simulink model "SF015A_WhlImbRejctn"  (R2013b)
settings: Solver=FixedStepDiscrete  SolverMode=SingleTasking  StartTime=0.0  StopTime=1  FixedStep=0.002  RelTol=1e-3
values from neighbouring files (symbols this model uses):
  ACTIVBANDMAX_ULS_U32 = DataDict.Constant    [SF015A_WhlImbRejctn_DataDict.m]
  ADAPVFILMAX_ULS_F32 = DataDict.Constant    [SF015A_WhlImbRejctn_DataDict.m]
  ARCHGLBPRM_180OVERPI_ULS_F32 = DataDict.Constant    [SF015A_WhlImbRejctn_DataDict.m]
  ARCHGLBPRM_2MILLISEC_SEC_F32 = DataDict.Constant    [SF015A_WhlImbRejctn_DataDict.m]
  ARCHGLBPRM_2PI_ULS_F32 = DataDict.Constant    [SF015A_WhlImbRejctn_DataDict.m]
  ARCHGLBPRM_FLOATZEROTHD_ULS_F32 = DataDict.Constant    [SF015A_WhlImbRejctn_DataDict.m]
  ARCHGLBPRM_PI_ULS_F32 = DataDict.Constant    [SF015A_WhlImbRejctn_DataDict.m]
  ARCHGLBPRM_PIOVER180_ULS_F32 = DataDict.Constant    [SF015A_WhlImbRejctn_DataDict.m]
  ARCHGLBPRM_PIOVER2_ULS_F32 = DataDict.Constant    [SF015A_WhlImbRejctn_DataDict.m]
  CALMINSPERCOUNT_ULS_F32 = DataDict.Constant    [SF015A_WhlImbRejctn_DataDict.m]
  DURATIONDISABLE_CNT_U16 = DataDict.Constant    [SF015A_WhlImbRejctn_DataDict.m]
  FILTWHLSPDMAX_MOTRADPERSEC_F32 = DataDict.Constant    [SF015A_WhlImbRejctn_DataDict.m]
  MICROSECTOMILLISEC_ULS_F32 = DataDict.Constant    [SF015A_WhlImbRejctn_DataDict.m]
  MINSTOMILLISEC_ULS_F32 = DataDict.Constant    [SF015A_WhlImbRejctn_DataDict.m]
  NINETY_ULS_F32 = DataDict.Constant    [SF015A_WhlImbRejctn_DataDict.m]
  NODEBSTEP_CNT_U16 = DataDict.Constant    [SF015A_WhlImbRejctn_DataDict.m]
  NROFDLY_CNT_U08 = DataDict.Constant    [SF015A_WhlImbRejctn_DataDict.m]
  ONEHALF_ULS_F32 = DataDict.Constant    [SF015A_WhlImbRejctn_DataDict.m]
  ONEHUNDRED_ULS_F32 = DataDict.Constant    [SF015A_WhlImbRejctn_DataDict.m]
  ONEOVRTHREE_ULS_F32 = DataDict.Constant    [SF015A_WhlImbRejctn_DataDict.m]
  ONEOVRTWENTY_ULS_F32 = DataDict.Constant    [SF015A_WhlImbRejctn_DataDict.m]
  ONETHOUSAND_ULS_F32 = DataDict.Constant    [SF015A_WhlImbRejctn_DataDict.m]
  PEAKMAX_ULS_F32 = DataDict.Constant    [SF015A_WhlImbRejctn_DataDict.m]
  PEAKMIN_ULS_F32 = DataDict.Constant    [SF015A_WhlImbRejctn_DataDict.m]
  PHAADJMAX_ULS_F32 = DataDict.Constant    [SF015A_WhlImbRejctn_DataDict.m]
  PITIMESSAMPLETIME_ULS_F32 = DataDict.Constant    [SF015A_WhlImbRejctn_DataDict.m]
  STOREDMINSPERCOUNT_ULS_F32 = DataDict.Constant    [SF015A_WhlImbRejctn_DataDict.m]
  TWO_ULS_F32 = DataDict.Constant    [SF015A_WhlImbRejctn_DataDict.m]
  TWOOVRTHREE_ULS_F32 = DataDict.Constant    [SF015A_WhlImbRejctn_DataDict.m]
  WhlImbRejctnAdpvFac = DataDict.Calibration    [SF015A_WhlImbRejctn_DataDict.m]
  WhlImbRejctnAutScaEna = DataDict.Calibration    [SF015A_WhlImbRejctn_DataDict.m]
  WhlImbRejctnAutScaTar = DataDict.Calibration    [SF015A_WhlImbRejctn_DataDict.m]
  WhlImbRejctnCurrMgnSlewPerLoop = DataDict.Calibration    [SF015A_WhlImbRejctn_DataDict.m]
  WhlImbRejctnDcTrendFltRcvryDly = DataDict.Calibration    [SF015A_WhlImbRejctn_DataDict.m]
  WhlImbRejctnDcTrendFltRcvryNegStep = DataDict.Calibration    [SF015A_WhlImbRejctn_DataDict.m]
  WhlImbRejctnDcTrendFltRcvryPosStep = DataDict.Calibration    [SF015A_WhlImbRejctn_DataDict.m]
  WhlImbRejctnDcTrendFltRcvryThd = DataDict.Calibration    [SF015A_WhlImbRejctn_DataDict.m]
  WhlImbRejctnDcTrendTh2Tq = DataDict.Calibration    [SF015A_WhlImbRejctn_DataDict.m]
  WhlImbRejctnDcTrendThTq = DataDict.Calibration    [SF015A_WhlImbRejctn_DataDict.m]
  WhlImbRejctnDcTrendTi2Sec = DataDict.Calibration    [SF015A_WhlImbRejctn_DataDict.m]
  WhlImbRejctnDcTrendTiSec = DataDict.Calibration    [SF015A_WhlImbRejctn_DataDict.m]
  WhlImbRejctnEnaSlewPerLoop = DataDict.Calibration    [SF015A_WhlImbRejctn_DataDict.m]
  WhlImbRejctnFctEna = DataDict.Calibration    [SF015A_WhlImbRejctn_DataDict.m]
  WhlImbRejctnFrqDiagcAmpThd = DataDict.Calibration    [SF015A_WhlImbRejctn_DataDict.m]
  WhlImbRejctnFrqDiagcEna = DataDict.Calibration    [SF015A_WhlImbRejctn_DataDict.m]
  WhlImbRejctnFrqDiagcFltRcvryDly = DataDict.Calibration    [SF015A_WhlImbRejctn_DataDict.m]
  WhlImbRejctnFrqDiagcFltRcvryNegStep = DataDict.Calibration    [SF015A_WhlImbRejctn_DataDict.m]
  WhlImbRejctnFrqDiagcFltRcvryPosStep = DataDict.Calibration    [SF015A_WhlImbRejctn_DataDict.m]
  WhlImbRejctnFrqDiagcFltRcvryThd = DataDict.Calibration    [SF015A_WhlImbRejctn_DataDict.m]
  WhlImbRejctnFrqDiagcThd = DataDict.Calibration    [SF015A_WhlImbRejctn_DataDict.m]
  WhlImbRejctnFrqDiagcTout = DataDict.Calibration    [SF015A_WhlImbRejctn_DataDict.m]
  WhlImbRejctnFrqDiagcUgrPoleMgn = DataDict.Calibration    [SF015A_WhlImbRejctn_DataDict.m]
  WhlImbRejctnFrqScaTblX = DataDict.Calibration    [SF015A_WhlImbRejctn_DataDict.m]
  WhlImbRejctnMaxDurn = DataDict.Calibration    [SF015A_WhlImbRejctn_DataDict.m]
  WhlImbRejctnMaxMgn = DataDict.Calibration    [SF015A_WhlImbRejctn_DataDict.m]
  WhlImbRejctnMaxMgnFltNegStep = DataDict.Calibration    [SF015A_WhlImbRejctn_DataDict.m]
  WhlImbRejctnMaxMgnFltPosStep = DataDict.Calibration    [SF015A_WhlImbRejctn_DataDict.m]
  WhlImbRejctnMaxMgnFltRcvryDly = DataDict.Calibration    [SF015A_WhlImbRejctn_DataDict.m]
  WhlImbRejctnMaxMgnFltRcvryNegStep = DataDict.Calibration    [SF015A_WhlImbRejctn_DataDict.m]
  WhlImbRejctnMaxMgnFltRcvryPosStep = DataDict.Calibration    [SF015A_WhlImbRejctn_DataDict.m]
  WhlImbRejctnMaxMgnFltRcvryThd = DataDict.Calibration    [SF015A_WhlImbRejctn_DataDict.m]
  WhlImbRejctnMaxMgnFltThd = DataDict.Calibration    [SF015A_WhlImbRejctn_DataDict.m]
  WhlImbRejctnMgnEstimnDeltaSca = DataDict.Calibration    [SF015A_WhlImbRejctn_DataDict.m]
  WhlImbRejctnMgnEstimnDiThd = DataDict.Calibration    [SF015A_WhlImbRejctn_DataDict.m]
  WhlImbRejctnMgnEstimnEnaThd = DataDict.Calibration    [SF015A_WhlImbRejctn_DataDict.m]
  WhlImbRejctnMgnEstimnFrq = DataDict.Calibration    [SF015A_WhlImbRejctn_DataDict.m]
  WhlImbRejctnMgnEstimnFrqDelta = DataDict.Calibration    [SF015A_WhlImbRejctn_DataDict.m]
  WhlImbRejctnMgnEstimnLeak = DataDict.Calibration    [SF015A_WhlImbRejctn_DataDict.m]
  WhlImbRejctnRampDwnTi = DataDict.Calibration    [SF015A_WhlImbRejctn_DataDict.m]
  WhlImbRejctnScaCncl = DataDict.Calibration    [SF015A_WhlImbRejctn_DataDict.m]
  WhlImbRejctnUgrPoleMgn = DataDict.Calibration    [SF015A_WhlImbRejctn_DataDict.m]
  WhlImbRejctnVehSpdEna = DataDict.Calibration    [SF015A_WhlImbRejctn_DataDict.m]
  WhlImbRejctnWhlSpdCorrlnFltRcvryDly = DataDict.Calibration    [SF015A_WhlImbRejctn_DataDict.m]
  WhlImbRejctnWhlSpdCorrlnFltRcvryNegStep = DataDict.Calibration    [SF015A_WhlImbRejctn_DataDict.m]
  WhlImbRejctnWhlSpdCorrlnFltRcvryPosStep = DataDict.Calibration    [SF015A_WhlImbRejctn_DataDict.m]
  WhlImbRejctnWhlSpdCorrlnFltRcvryThd = DataDict.Calibration    [SF015A_WhlImbRejctn_DataDict.m]
  WhlImbRejctnWhlSpdCorrlnThd = DataDict.Calibration    [SF015A_WhlImbRejctn_DataDict.m]
  WhlImbRejctnWhlSpdCorrlnTi = DataDict.Calibration    [SF015A_WhlImbRejctn_DataDict.m]
  WIRCMDMAX_MOTNWTMTR_F32 = DataDict.Constant    [SF015A_WhlImbRejctn_DataDict.m]
  ZERO_ULS_F32 = DataDict.Constant    [SF015A_WhlImbRejctn_DataDict.m]
undefined symbols (not defined in the file or in its folder): Cntr, NtcNr1, NvmGetErrSts1, SigQlfr1, Sts, SysSt1
libraries: simulink x32, FixdToFloat x32, Fil x20, NxtrLim x15, NxtrNvM x12, NxtrAbslt x8, NxtrMath x7, NxtrMax x6, NxtrMin x4, FloatToFixd x2, LnrIntrpn x2, NxtrSign x1
(part 4 of 12)

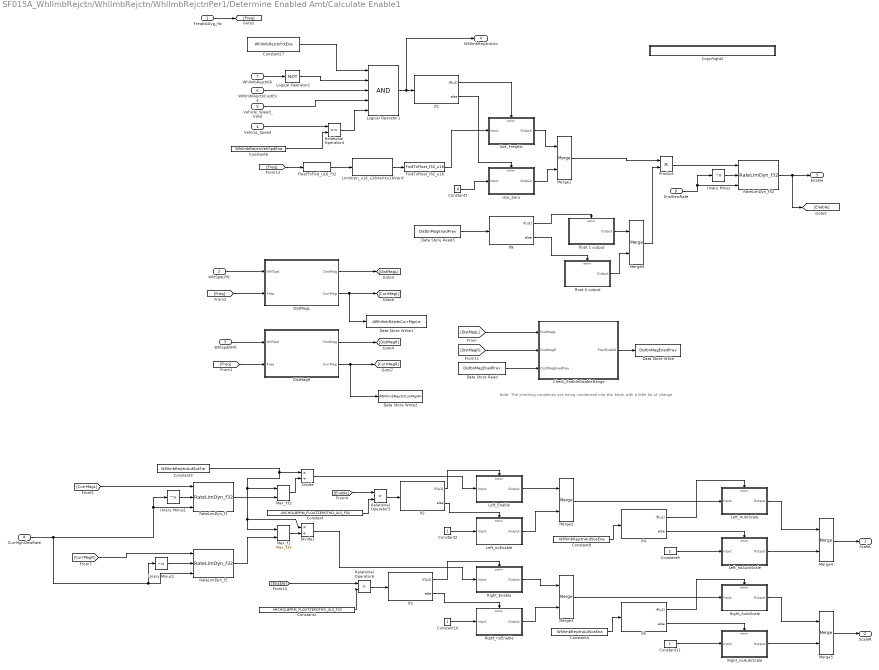
== system SF015A_WhlImbRejctn/WhlImbRejctn/WhlImbRejctnPer1/Determine Enabled Amt/Calculate Enable1 ==
  note: Note: The checking conditions are being condensed into thsi block with a little bit of change
  FreqEstAvg_Hz : Inport
  WhlSpdLFilt : Inport  Port=2
  WhlSpdRFilt : Inport  Port=3
  Vehicle_Speed : Inport  Port=4
  Vehicle_Speed_Valid : Inport  Port=5
  WhlImbRejctnCustEna : Inport  Port=6
  WhlImbRejctnDi : Inport  Port=7
  CurrMgnSlewRate : Inport  Port=8
  EnaSlewRate : Inport  Port=9
  Check_EnableDisableRange : Subsystem
  Constant : Constant  Value=ARCHGLBPRM_FLOATZEROTHD_ULS_F32
  Constant1 : Constant  Value=ARCHGLBPRM_FLOATZEROTHD_ULS_F32
  Constant{2,9..11} (4 alike) : Constant  OutDataTypeStr=single
  Constant17 : Constant  Value=WhlImbRejctnFctEna
  Constant3 : Constant  Value=WhlImbRejctnAutScaTar
  Constant4 : Constant  Value=WhlImbRejctnAutScaEna
  Constant6 : Constant  Value=WhlImbRejctnVehSpdEna
  Constant7 : Constant  Value=0  OutDataTypeStr=single
  Constant8 : Constant  Value=WhlImbRejctnAutScaEna
  CopyRight2 : Subsystem  Description=|  mask(Copyright Information){none=on}
      | Copyright info block.                                               
      |                                                                     
      | Place copyright information at the top of every subsystem in design.
      mask prompts: none "No parameters"
      mask help: Place copyright information at the top of every subsystem in design.
      mask Display:
      | NxtrConf = 'Nexteer Confidential';
      | 
      | sys = bdroot; %handle for the current model ("system")
      | first = get_param(sys,'Created');
      | first = first(end-3:end);  %year is last four digits
      | 
      | last = get_param(sys,'LastModifiedDate');
      | if isempty(last)
      |     last = datestr(now,'yyyy');
      | else
      |     last = last(end-3:end);
      | end
      | 
      | if strcmp(first,last)
      |     fprintf('%s -- Copyright %s Nexteer',NxtrConf,first)
      | else
      |     fprintf('%s -- %s%s- %s Nexteer',NxtrConf,char(169),first,last)
      | end
  Data Store Read : DataStoreRead  Priority=2  DataStoreName=DistbnMagEnadPrev
      settings: AttributesFormatString=Priority=%<Priority>
  Data Store Read3 : DataStoreRead  Priority=1  DataStoreName=DistbnMagEnadPrev
      settings: AttributesFormatString=Priority=%<Priority>
  Data Store Write : DataStoreWrite  Priority=3  DataStoreName=DistbnMagEnadPrev
      settings: AttributesFormatString=Priority=%<Priority>
  Data Store Write1 : DataStoreWrite  DataStoreName=dWhlImbRejctnCurrMgnLe
  Data Store Write2 : DataStoreWrite  DataStoreName=dWhlImbRejctnCurrMgnRi
  DistMagL : Subsystem
  DistMagR : Subsystem
  Divide : Product  Inputs=*/
  Divide1 : Product  Inputs=*/
  FixdToFloat_f32_u16 : FixdToFloat/FixdToFloat_f32_u16  Param1=0
  FloatToFixd_u16_f32 : FloatToFixd/FloatToFixd_u16_f32  Param1=0
  If1 : If  RequirementInfo={} %GIDa_7d8297b8_b265_4b47_b8b2_192e5a92e4fb  IfExpression=u1
  If2 : If  RequirementInfo={} %GIDa_0556d171_7866_4516_8d40_956f321be7bc  IfExpression=u1
  If3 : If  RequirementInfo={} %GIDa_fcbce161_0599_4b7a_b23c_d7b8d7e27a0f  IfExpression=u1
  If4 : If  RequirementInfo={} %GIDa_46a5a10e_d4b7_40a4_ac58_d797cb624c83  IfExpression=u1
  If5 : If  RequirementInfo={} %GIDa_3e7d8d50_75ba_4493_bb61_e3ba5f1e5c7c  IfExpression=u1
  If9 : If  RequirementInfo={} %GIDa_220c56c6_5b09_48da_a4b3_63431d3edf67  IfExpression=u1
  Left_AutoScale : Subsystem  RequirementInfo={} %GIDa_9c3ac42f_cbc1_49be_98f6_7ec1737ed2ed  TreatAsAtomicUnit=on
  Left_Enable : Subsystem  RequirementInfo={} %GIDa_d65479b8_5b54_4e68_bf36_3b31ad24537e  TreatAsAtomicUnit=on
  Left_noAutoScale : Subsystem  RequirementInfo={} %GIDa_bdc4660b_a72c_40f0_89ba_28a8acc1db11  TreatAsAtomicUnit=on
  Left_noEnable : Subsystem  RequirementInfo={} %GIDa_18e28b2f_1f1d_4076_8343_147cb5570336  TreatAsAtomicUnit=on
  LnrIntrpn_u16_u16VariXu16VariY : LnrIntrpn/LnrIntrpn_u16_u16VariXu16VariY  XTbl=WhlImbRejctnFrqScaTblX  YTbl=WhlImbRejctnFrqScaTblY
      settings: AttributesFormatString=Lnr ( u16VariX , u16VariY )
  Logical Operator1 : Logic  Inputs=5  AllPortsSameDT=off  OutDataTypeStr=boolean
  Logical Operator2 : Logic  Operator=NOT  Inputs=5  AllPortsSameDT=off  OutDataTypeStr=boolean
  Max_f1 : NxtrMax/Max_f32  SFunctionSpec=single y1 = Max_f32(single u1, single u2)
      settings: AttributesFormatString=%<Name>
  Max_f32 : NxtrMax/Max_f32  SFunctionSpec=single y1 = Max_f32(single u1, single u2)
      settings: AttributesFormatString=%<Name>
  Merge{1..5,9} (6 alike) : Merge
  Product : Product
  RateLimDyn_f1 : NxtrLim/RateLimDyn_f32  StVar=LeCurrMgnSlewPerLoop  Ts=ARCHGLBPRM_2MILLISEC_SEC_F32
      settings: AttributesFormatString=StVar: %<StVar>
  RateLimDyn_f2 : NxtrLim/RateLimDyn_f32  StVar=RiCurrMgnSlewPerLoop  Ts=ARCHGLBPRM_2MILLISEC_SEC_F32
      settings: AttributesFormatString=StVar: %<StVar>
  RateLimDyn_f32 : NxtrLim/RateLimDyn_f32  StVar=EnaSlewPerLoop  Ts=ARCHGLBPRM_2MILLISEC_SEC_F32
      settings: AttributesFormatString=StVar: %<StVar>
  Relational Operator4 : RelationalOperator  OutDataTypeStr=boolean
  Relational Operator5 : RelationalOperator  Operator=>  OutDataTypeStr=boolean
  Relational Operator6 : RelationalOperator  Operator=>  OutDataTypeStr=boolean
  Right_AutoScale : Subsystem  RequirementInfo={} %GIDa_13da9aa5_5c49_428f_b287_6188729282ed  TreatAsAtomicUnit=on
  Right_Enable : Subsystem  RequirementInfo={} %GIDa_75bbbddb_2767_47a3_9165_63797ed0e216  TreatAsAtomicUnit=on
  Right_noAutoScale : Subsystem  RequirementInfo={} %GIDa_e3eec680_517e_4da7_948a_b3f8124b2971  TreatAsAtomicUnit=on
  Right_noEnable : Subsystem  RequirementInfo={} %GIDa_b2607bc0_d58b_406c_8b11_3dee4f11cd4c  TreatAsAtomicUnit=on
  Unary Minus : UnaryMinus
  Unary Minus1 : UnaryMinus
  Unary Minus2 : UnaryMinus
  Use_FreqEst : Subsystem  RequirementInfo={} %GIDa_066b3e73_a3fa_4d6c_9937_967fb698f328  TreatAsAtomicUnit=on
  Use_Zero : Subsystem  RequirementInfo={} %GIDa_7b829dcd_761e_44e8_86d6_74abc0632468  TreatAsAtomicUnit=on
  float 0 output : Subsystem  RequirementInfo={} %GIDa_73b9442c_5069_415a_a71a_08570183037e  TreatAsAtomicUnit=on
  float 1 output : Subsystem  RequirementInfo={} %GIDa_eb48623e_e509_47ed_bd29_5bcb251c6a65  TreatAsAtomicUnit=on
  ScaleL : Outport
  ScaleR : Outport  Port=2
  Enable : Outport  Port=3
  WhlImbRejctnActv : Outport  Port=4
  wires:
  FreqEstAvg_Hz/1 -> [Freq]
  WhlSpdLFilt/1 -> DistMagL/1(WhlSpd)
  [Freq] -> DistMagL/2(Freq)
  WhlSpdRFilt/1 -> DistMagR/1(WhlSpd)
  [Freq] -> DistMagR/2(Freq)
  DistMagL/1(DistMag) -> [DistMagL]
  DistMagR/1(DistMag) -> [DistMagR]
  Data Store Read3/1 -> If9/1
  Constant3/1 -> Max_f32/1, Max_f1/1, Divide1/1, Divide/1
  DistMagL/2(CurrMag) -> Data Store Write1/1, [CurrMagL]
  DistMagR/2(CurrMag) -> Data Store Write2/1, [CurrMagR]
  Max_f32/1 -> Divide/2
  [CurrMagL] -> RateLimDyn_f1/1
  Max_f1/1 -> Divide1/2
  [CurrMagR] -> RateLimDyn_f2/1
  Vehicle_Speed/1 -> Relational Operator4/1
  Constant6/1 -> Relational Operator4/2
  Relational Operator4/1 -> Logical Operator1/5
  Vehicle_Speed_Valid/1 -> Logical Operator1/4
  WhlImbRejctnCustEna/1 -> Logical Operator1/3
  WhlImbRejctnDi/1 -> Logical Operator2/1
  Constant7/1 -> Use_Zero/1(Input)
  If1/1 -> Use_FreqEst/Action
  If1/2 -> Use_Zero/Action
  Logical Operator1/1 -> WhlImbRejctnActv/1, If1/1
  Use_FreqEst/1(Output) -> Merge1/1
  Use_Zero/1(Output) -> Merge1/2
  Merge1/1 -> Product/1
  [Freq] -> FloatToFixd_u16_f32/1
  FixdToFloat_f32_u16/1 -> Use_FreqEst/1(Input)
  LnrIntrpn_u16_u16VariXu16VariY/1 -> FixdToFloat_f32_u16/1
  FloatToFixd_u16_f32/1 -> LnrIntrpn_u16_u16VariXu16VariY/1
  Product/1 -> RateLimDyn_f32/1
  Constant2/1 -> Left_noEnable/1(Input)
  If2/1 -> Left_Enable/Action
  If2/2 -> Left_noEnable/Action
  Left_Enable/1(Output) -> Merge2/1
  Left_noEnable/1(Output) -> Merge2/2
  Divide/1 -> Left_Enable/1(Input)
  [Enable] -> Relational Operator5/1
  Constant10/1 -> Right_noEnable/1(Input)
  If3/1 -> Right_Enable/Action
  If3/2 -> Right_noEnable/Action
  Right_Enable/1(Output) -> Merge3/1
  Right_noEnable/1(Output) -> Merge3/2
  Divide1/1 -> Right_Enable/1(Input)
  If4/1 -> Left_AutoScale/Action
  If4/2 -> Left_noAutoScale/Action
  Left_AutoScale/1(Output) -> Merge4/1
  Left_noAutoScale/1(Output) -> Merge4/2
  Merge2/1 -> Left_AutoScale/1(Input)
  Constant8/1 -> If4/1
  Merge4/1 -> ScaleL/1
  Constant9/1 -> Left_noAutoScale/1(Input)
  If5/1 -> Right_AutoScale/Action
  If5/2 -> Right_noAutoScale/Action
  Right_AutoScale/1(Output) -> Merge5/1
  Right_noAutoScale/1(Output) -> Merge5/2
  Merge3/1 -> Right_AutoScale/1(Input)
  Constant4/1 -> If5/1
  Constant11/1 -> Right_noAutoScale/1(Input)
  Merge5/1 -> ScaleR/1
  RateLimDyn_f32/1 -> Enable/1, [Enable]
  Unary Minus/1 -> RateLimDyn_f32/2
  Unary Minus1/1 -> RateLimDyn_f1/2
  RateLimDyn_f1/1 -> Max_f32/2
  CurrMgnSlewRate/1 -> RateLimDyn_f2/3, Unary Minus2/1, Unary Minus1/1, RateLimDyn_f1/3
  Unary Minus2/1 -> RateLimDyn_f2/2
  RateLimDyn_f2/1 -> Max_f1/2
  Constant17/1 -> Logical Operator1/1
  Merge9/1 -> Product/2
  Relational Operator5/1 -> If2/1
  Relational Operator6/1 -> If3/1
  EnaSlewRate/1 -> RateLimDyn_f32/3, Unary Minus/1
  Constant/1 -> Relational Operator5/2
  [Enable] -> Relational Operator6/1
  Constant1/1 -> Relational Operator6/2
  If9/1 -> float 1 output/Action
  float 1 output/1(Output) -> Merge9/1
  If9/2 -> float 0 output/Action
  float 0 output/1(Output) -> Merge9/2
  Logical Operator2/1 -> Logical Operator1/2
  [DistMagL] -> Check_EnableDisableRange/1(DistMagL)
  [DistMagR] -> Check_EnableDisableRange/2(DistMagR)
  Data Store Read/1 -> Check_EnableDisableRange/3(DistMagEnadPrev)
  Check_EnableDisableRange/1(PrevEnabld) -> Data Store Write/1

== system SF015A_WhlImbRejctn/WhlImbRejctn/WhlImbRejctnPer1/Determine Enabled Amt/CopyRight2 ==

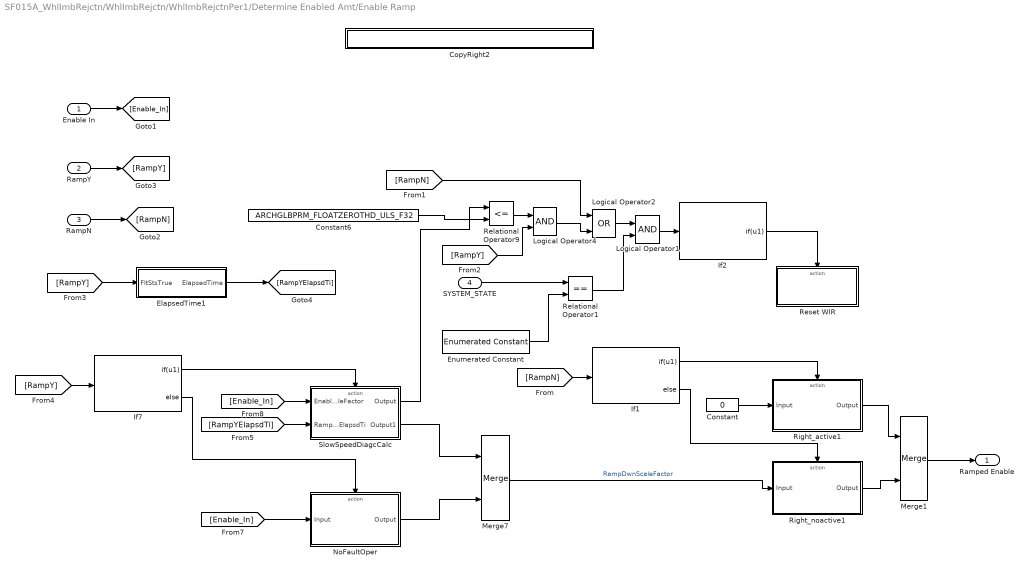
== system SF015A_WhlImbRejctn/WhlImbRejctn/WhlImbRejctnPer1/Determine Enabled Amt/Enable Ramp ==
  Enable In : Inport
  "RampY " : Inport  Port=2
  RampN : Inport  Port=3
  SYSTEM_STATE : Inport  Port=4
  Constant : Constant  Value=0  OutDataTypeStr=single
  Constant6 : Constant  Value=ARCHGLBPRM_FLOATZEROTHD_ULS_F32
  CopyRight2 : Subsystem  Description=|  mask(Copyright Information){none=on}
      | Copyright info block.                                               
      |                                                                     
      | Place copyright information at the top of every subsystem in design.
      mask prompts: none "No parameters"
      mask help: Place copyright information at the top of every subsystem in design.
      mask Display:
      | NxtrConf = 'Nexteer Confidential';
      | 
      | sys = bdroot; %handle for the current model ("system")
      | first = get_param(sys,'Created');
      | first = first(end-3:end);  %year is last four digits
      | 
      | last = get_param(sys,'LastModifiedDate');
      | if isempty(last)
      |     last = datestr(now,'yyyy');
      | else
      |     last = last(end-3:end);
      | end
      | 
      | if strcmp(first,last)
      |     fprintf('%s -- Copyright %s Nexteer',NxtrConf,first)
      | else
      |     fprintf('%s -- %s%s- %s Nexteer',NxtrConf,char(169),first,last)
      | end
  ElapsedTime1 : Subsystem  TreatAsAtomicUnit=on
  Enumerated Constant : simulink/Sources/Enumerated Constant  OutDataTypeStr=Enum: SysSt1  Value=SysSt1.SYSST_ENA  SampleTime=inf
  If1 : If  RequirementInfo={} %GIDa_bfd6920b_006a_416f_b6f7_6ef0775419c8  IfExpression=u1
  If2 : If  RequirementInfo={} %GIDa_894989e0_ef65_43c4_bfdb_f22d51c8efad  IfExpression=u1  ShowElse=off
  If7 : If  RequirementInfo={} %GIDa_516cf2d0_a63b_46fe_b255_3d41307786bb  IfExpression=u1
  Logical Operator1 : Logic  AllPortsSameDT=off  OutDataTypeStr=boolean
  Logical Operator2 : Logic  Operator=OR  AllPortsSameDT=off  OutDataTypeStr=boolean
  Logical Operator4 : Logic  AllPortsSameDT=off  OutDataTypeStr=boolean
  Merge1 : Merge
  Merge7 : Merge
  NoFaultOper : Subsystem  RequirementInfo={} %GIDa_85bb45c8_b5a9_4bce_b96d_1bcc95564bc7  TreatAsAtomicUnit=on
  Relational Operator1 : RelationalOperator  Operator===  OutDataTypeStr=boolean
  Relational Operator9 : RelationalOperator  Operator=<=  OutDataTypeStr=boolean
  "Reset WIR " : Subsystem  TreatAsAtomicUnit=on
  Right_active1 : Subsystem  RequirementInfo={} %GIDa_d211d460_285e_47ce_a10a_276eb1a21d5a  TreatAsAtomicUnit=on
  Right_noactive1 : Subsystem  RequirementInfo={} %GIDa_3ffdf98d_b314_4708_8422_325b4c42ba1c  TreatAsAtomicUnit=on
  SlowSpeedDiagcCalc : Subsystem  RequirementInfo={} %GIDa_b7c7be65_73bf_45a8_bfe0_fa96a024938d  TreatAsAtomicUnit=on
  Ramped Enable : Outport
  wires:
  Constant6/1 -> Relational Operator9/2
  Relational Operator9/1 -> Logical Operator4/1
  Logical Operator4/1 -> Logical Operator2/2
  Logical Operator1/1 -> If2/1
  Enable In/1 -> [Enable_In]
  "RampY "/1 -> [RampY]
  [RampN] -> Logical Operator2/1
  If7/1 -> SlowSpeedDiagcCalc/Action
  If7/2 -> NoFaultOper/Action
  NoFaultOper/1(Output) -> Merge7/2
  [Enable_In] -> NoFaultOper/1(Input)
  If1/1 -> Right_active1/Action
  If1/2 -> Right_noactive1/Action
  Right_active1/1(Output) -> Merge1/1
  Right_noactive1/1(Output) -> Merge1/2
  Merge7/1 -> Right_noactive1/1(Input)  "RampDwnScaleFactor"
  Constant/1 -> Right_active1/1(Input)
  [RampN] -> If1/1
  Merge1/1 -> Ramped Enable/1
  [Enable_In] -> SlowSpeedDiagcCalc/1(EnableScaleFactor)
  RampN/1 -> [RampN]
  [RampY] -> Logical Operator4/2
  [RampYElapsdTi] -> SlowSpeedDiagcCalc/2(RampYElapsdTi)
  [RampY] -> If7/1
  If2/1 -> "Reset WIR "/Action
  SYSTEM_STATE/1 -> Relational Operator1/1
  Enumerated Constant/1 -> Relational Operator1/2
  Logical Operator2/1 -> Logical Operator1/1
  Relational Operator1/1 -> Logical Operator1/2
  SlowSpeedDiagcCalc/1(Output) -> Relational Operator9/1
  SlowSpeedDiagcCalc/2(Output1) -> Merge7/1
  [RampY] -> ElapsedTime1/1(FltStsTrue)
  ElapsedTime1/1(ElapsedTime) -> [RampYElapsdTi]

== system SF015A_WhlImbRejctn/WhlImbRejctn/WhlImbRejctnPer1/WIR Diagnostics/Amplitude Calculation1 ==
  Input : Inport
  Abslt_f32_f32 : NxtrAbslt/Abslt_f32_f32  SFunctionSpec=single y1 = Abslt_f32_f32(single u1)
      settings: AttributesFormatString=%<Name>
  Constant : Constant  Value=ARCHGLBPRM_PIOVER2_ULS_F32
  CopyRight2 : Subsystem  Description=|  mask(Copyright Information){none=on}
      | Copyright info block.                                               
      |                                                                     
      | Place copyright information at the top of every subsystem in design.
      mask prompts: none "No parameters"
      mask help: Place copyright information at the top of every subsystem in design.
      mask Display:
      | NxtrConf = 'Nexteer Confidential';
      | 
      | sys = bdroot; %handle for the current model ("system")
      | first = get_param(sys,'Created');
      | first = first(end-3:end);  %year is last four digits
      | 
      | last = get_param(sys,'LastModifiedDate');
      | if isempty(last)
      |     last = datestr(now,'yyyy');
      | else
      |     last = last(end-3:end);
      | end
      | 
      | if strcmp(first,last)
      |     fprintf('%s -- Copyright %s Nexteer',NxtrConf,first)
      | else
      |     fprintf('%s -- %s%s- %s Nexteer',NxtrConf,char(169),first,last)
      | end
  FilLpUpdOutp : Fil/FilLpUpdOutp  StVar=BlndCmdMgnLp1Fil
      settings: AttributesFormatString=StVar: %<StVar>
  FilLpUpdOutp1 : Fil/FilLpUpdOutp  StVar=BlndCmdMgnLp2Fil
      settings: AttributesFormatString=StVar: %<StVar>
  Product : Product
  Amp : Outport
  wires:
  FilLpUpdOutp1/1 -> Amp/1
  FilLpUpdOutp/1 -> Product/1
  Abslt_f32_f32/1 -> FilLpUpdOutp/1
  Input/1 -> Abslt_f32_f32/1
  Product/1 -> FilLpUpdOutp1/1
  Constant/1 -> Product/2

== system SF015A_WhlImbRejctn/WhlImbRejctn/WhlImbRejctnPer1/WIR Diagnostics/CopyRight2 ==

== system SF015A_WhlImbRejctn/WhlImbRejctn/WhlImbRejctnPer1/WIR Diagnostics/DcTrendDiag ==
  WIRCmd : Inport
  Abslt_f32_f32 : NxtrAbslt/Abslt_f32_f32  SFunctionSpec=single y1 = Abslt_f32_f32(single u1)
      settings: AttributesFormatString=%<Name>
  Constant : Constant  Value=ONETHOUSAND_ULS_F32
  Constant1 : Constant  Value=ONETHOUSAND_ULS_F32
  Constant13 : Constant  Value=0  OutDataTypeStr=boolean
  Constant2 : Constant  OutDataTypeStr=Inherit: Inherit via back propagation
  Constant3 : Constant  Value=WhlImbRejctnDcTrendTi2Sec
  Constant4 : Constant  Value=WhlImbRejctnDcTrendThTq
  Constant5 : Constant  Value=WhlImbRejctnDcTrendTiSec
  Constant6 : Constant  Value=WhlImbRejctnDcTrendTh2Tq
  CopyRight2 : Subsystem  Description=|  mask(Copyright Information){none=on}
      | Copyright info block.                                               
      |                                                                     
      | Place copyright information at the top of every subsystem in design.
      mask prompts: none "No parameters"
      mask help: Place copyright information at the top of every subsystem in design.
      mask Display:
      | NxtrConf = 'Nexteer Confidential';
      | 
      | sys = bdroot; %handle for the current model ("system")
      | first = get_param(sys,'Created');
      | first = first(end-3:end);  %year is last four digits
      | 
      | last = get_param(sys,'LastModifiedDate');
      | if isempty(last)
      |     last = datestr(now,'yyyy');
      | else
      |     last = last(end-3:end);
      | end
      | 
      | if strcmp(first,last)
      |     fprintf('%s -- Copyright %s Nexteer',NxtrConf,first)
      | else
      |     fprintf('%s -- %s%s- %s Nexteer',NxtrConf,char(169),first,last)
      | end
  DCTrendFault : Subsystem  RequirementInfo={} %GIDa_a2bf172f_152a_4264_a2d8_48cf318cb81e  TreatAsAtomicUnit=on
  Data Type Conversion : DataTypeConversion  OutDataTypeStr=boolean
  Data Type Conversion1 : DataTypeConversion  OutDataTypeStr=boolean
  ElapsedTime1 : Subsystem  TreatAsAtomicUnit=on
  ElapsedTime2 : Subsystem  TreatAsAtomicUnit=on
  FilLpUpdOutp : Fil/FilLpUpdOutp  StVar=DcTrendLpFil
      settings: AttributesFormatString=StVar: %<StVar>
  If5 : If  RequirementInfo={} %GIDa_0ecf552f_0a22_4e50_8225_2e691f1dcd0f  IfExpression=u1
  Logical Operator1 : Logic  Operator=OR  AllPortsSameDT=off  OutDataTypeStr=boolean
  Merge5 : Merge
  NoFault : Subsystem  RequirementInfo={} %GIDa_b91ed932_8d0a_4501_94cd_eecd5662fa49  TreatAsAtomicUnit=on
  Product : Product
  Product1 : Product
  Relational Operator{1..4} (4 alike) : RelationalOperator  OutDataTypeStr=boolean
  FltStat : Outport
  wires:
  Merge5/1 -> FltStat/1
  Abslt_f32_f32/1 -> FilLpUpdOutp/1
  FilLpUpdOutp/1 -> Relational Operator1/1, Relational Operator3/1
  Constant4/1 -> Relational Operator1/2
  Relational Operator1/1 -> ElapsedTime1/1(FltStsTrue)
  ElapsedTime1/1(ElapsedTime) -> Relational Operator2/1
  Relational Operator3/1 -> ElapsedTime2/1(FltStsTrue)
  Constant3/1 -> Product/1
  Constant6/1 -> Relational Operator3/2
  Logical Operator1/1 -> If5/1
  Relational Operator4/1 -> Logical Operator1/1
  Relational Operator2/1 -> Logical Operator1/2
  If5/1 -> DCTrendFault/Action
  If5/2 -> NoFault/Action
  DCTrendFault/1(Output) -> Merge5/1
  NoFault/1(Output) -> Merge5/2
  Constant2/1 -> Data Type Conversion/1
  Constant13/1 -> Data Type Conversion1/1
  WIRCmd/1 -> Abslt_f32_f32/1
  Data Type Conversion/1 -> DCTrendFault/1(Input)
  Data Type Conversion1/1 -> NoFault/1(Input)
  ElapsedTime2/1(ElapsedTime) -> Relational Operator4/1
  Constant/1 -> Product/2
  Product/1 -> Relational Operator4/2
  Constant1/1 -> Product1/2
  Product1/1 -> Relational Operator2/2
  Constant5/1 -> Product1/1

== system SF015A_WhlImbRejctn/WhlImbRejctn/WhlImbRejctnPer1/WIR Diagnostics/FrequencyDiag ==
  WIRCmd : Inport
  FreqEst : Inport  Port=2
  Enable : Inport  Port=3
  CmdAmp : Inport  Port=4
  Constant1 : Constant  Value=0  OutDataTypeStr=boolean
  Constant13 : Constant  Value=0  OutDataTypeStr=boolean
  Constant2 : Constant  OutDataTypeStr=boolean
  Constant5 : Constant  Value=WhlImbRejctnFrqDiagcEna
  CopyRight2 : Subsystem  Description=|  mask(Copyright Information){none=on}
      | Copyright info block.                                               
      |                                                                     
      | Place copyright information at the top of every subsystem in design.
      mask prompts: none "No parameters"
      mask help: Place copyright information at the top of every subsystem in design.
      mask Display:
      | NxtrConf = 'Nexteer Confidential';
      | 
      | sys = bdroot; %handle for the current model ("system")
      | first = get_param(sys,'Created');
      | first = first(end-3:end);  %year is last four digits
      | 
      | last = get_param(sys,'LastModifiedDate');
      | if isempty(last)
      |     last = datestr(now,'yyyy');
      | else
      |     last = last(end-3:end);
      | end
      | 
      | if strcmp(first,last)
      |     fprintf('%s -- Copyright %s Nexteer',NxtrConf,first)
      | else
      |     fprintf('%s -- %s%s- %s Nexteer',NxtrConf,char(169),first,last)
      | end
  Data Type Conversion : DataTypeConversion  OutDataTypeStr=boolean
  Data Type Conversion1 : DataTypeConversion  OutDataTypeStr=boolean
  EnableDiag : Subsystem  RequirementInfo={} %GIDa_e70893fa_b476_41fc_83f3_cd56d2261539  TreatAsAtomicUnit=on
  FreqDiagFault : Subsystem  RequirementInfo={} %GIDa_823acb2c_63d2_4f8b_8737_5bdfc9749030  TreatAsAtomicUnit=on
  If1 : If  RequirementInfo={} %GIDa_84d76f80_37f5_41d4_ac0a_c93962678a05  IfExpression=u1
  If5 : If  RequirementInfo={} %GIDa_329d3e5e_6fe7_4407_98ef_92a7d72cbf0a  IfExpression=u1
  Merge1 : Merge
  Merge5 : Merge
  NoDiag : Subsystem  RequirementInfo={} %GIDa_2b829a4a_b804_4dfa_be7f_b9930fa6303f  TreatAsAtomicUnit=on
  NoFault : Subsystem  RequirementInfo={} %GIDa_4cd1cae6_1247_413b_bca5_d0a1fdb2931d  TreatAsAtomicUnit=on
  FltStat : Outport
  wires:
  Merge5/1 -> FltStat/1
  WIRCmd/1 -> EnableDiag/3(WIRCmd)
  FreqEst/1 -> EnableDiag/2(FreqEst)
  Enable/1 -> EnableDiag/4(Enable)
  Constant5/1 -> If1/1
  Merge1/1 -> If5/1
  CmdAmp/1 -> EnableDiag/1(WIRCmdAmp)
  If5/1 -> FreqDiagFault/Action
  If5/2 -> NoFault/Action
  FreqDiagFault/1(Output) -> Merge5/1
  NoFault/1(Output) -> Merge5/2
  Constant2/1 -> Data Type Conversion/1
  Constant13/1 -> Data Type Conversion1/1
  If1/1 -> EnableDiag/Action
  If1/2 -> NoDiag/Action
  EnableDiag/1(Output) -> Merge1/1
  NoDiag/1(Output) -> Merge1/2
  Constant1/1 -> NoDiag/1(Input)
  Data Type Conversion/1 -> FreqDiagFault/1(Input)
  Data Type Conversion1/1 -> NoFault/1(Input)

== system SF015A_WhlImbRejctn/WhlImbRejctn/WhlImbRejctnPer1/WIR Diagnostics/MaxMagDiag ==
  CmdAmp : Inport
  CopyRight2 : Subsystem  Description=|  mask(Copyright Information){none=on}
      | Copyright info block.                                               
      |                                                                     
      | Place copyright information at the top of every subsystem in design.
      mask prompts: none "No parameters"
      mask help: Place copyright information at the top of every subsystem in design.
      mask Display:
      | NxtrConf = 'Nexteer Confidential';
      | 
      | sys = bdroot; %handle for the current model ("system")
      | first = get_param(sys,'Created');
      | first = first(end-3:end);  %year is last four digits
      | 
      | last = get_param(sys,'LastModifiedDate');
      | if isempty(last)
      |     last = datestr(now,'yyyy');
      | else
      |     last = last(end-3:end);
      | end
      | 
      | if strcmp(first,last)
      |     fprintf('%s -- Copyright %s Nexteer',NxtrConf,first)
      | else
      |     fprintf('%s -- %s%s- %s Nexteer',NxtrConf,char(169),first,last)
      | end
  Magnitude Comparison : Subsystem
  FltStat : Outport
  wires:
  CmdAmp/1 -> Magnitude Comparison/1(WIRCmdAmp1)
  Magnitude Comparison/1(MagDiag) -> FltStat/1

== system SF015A_WhlImbRejctn/WhlImbRejctn/WhlImbRejctnPer1/WIR Diagnostics/Set NTC Block ==
  note: Logic for setting of NTC bit based on WheelFrequencyValid
      | signal has been removed.
  MaxMag : Inport
  DC Trend : Inport  Port=2
  FrqDiagc : Inport  Port=3
  WhlSpdCorrln : Inport  Port=4
  MaxPersis : Inport  Port=5
  Action Port : ActionPort  ActionType=then
  Bitwise Operator : simulink/Logic and Bit Operations/Bitwise Operator  logicop=OR  UseBitMask=off  NumInputPorts=5  BitMask=bin2dec('11011001')  BitMaskRealWorld=Stored Integer
  Constant11 : Constant  Value=NODEBSTEP_CNT_U16
  CopyRight2 : Subsystem  Description=|  mask(Copyright Information){none=on}
      | Copyright info block.                                               
      |                                                                     
      | Place copyright information at the top of every subsystem in design.
      mask prompts: none "No parameters"
      mask help: Place copyright information at the top of every subsystem in design.
      mask Display:
      | NxtrConf = 'Nexteer Confidential';
      | 
      | sys = bdroot; %handle for the current model ("system")
      | first = get_param(sys,'Created');
      | first = first(end-3:end);  %year is last four digits
      | 
      | last = get_param(sys,'LastModifiedDate');
      | if isempty(last)
      |     last = datestr(now,'yyyy');
      | else
      |     last = last(end-3:end);
      | end
      | 
      | if strcmp(first,last)
      |     fprintf('%s -- Copyright %s Nexteer',NxtrConf,first)
      | else
      |     fprintf('%s -- %s%s- %s Nexteer',NxtrConf,char(169),first,last)
      | end
  Enumerated Constant10 : simulink/Sources/Enumerated Constant  OutDataTypeStr=Enum: SigQlfr1  Value=SigQlfr1.SIGQLFR_FAILD  SampleTime=inf
  NTC Bit parameter info : Subsystem
  NTC Bit parameter info2 : Subsystem
  NTC Bit parameter info3 : Subsystem
  NTC Bit parameter info4 : Subsystem
  NTC Bit parameter info5 : Subsystem
  SetNtcSts : Subsystem  RequirementInfo={} %GIDa_b927cdae_753d_4a83_ad1f_c59a8153411f  TreatAsAtomicUnit=on
      settings: RTWSystemCode=Inline
  WirFltNtc : simulink/Sources/Enumerated Constant  OutDataTypeStr=Enum: NtcNr1  Value=NtcNr1.NTCNR_0X0A5  SampleTime=inf
  wires:
  DC Trend/1 -> NTC Bit parameter info2/1(Flag)
  FrqDiagc/1 -> NTC Bit parameter info3/1(Flag)
  WhlSpdCorrln/1 -> NTC Bit parameter info4/1(Flag)
  Bitwise Operator/1 -> SetNtcSts/2(NtcStInfo)
  WirFltNtc/1 -> SetNtcSts/1(NtcNr)
  Enumerated Constant10/1 -> SetNtcSts/3(NtcSts)
  Constant11/1 -> SetNtcSts/4(DebStep)
  MaxMag/1 -> NTC Bit parameter info/1(Flag)
  NTC Bit parameter info/1(FltBit) -> Bitwise Operator/1
  MaxPersis/1 -> NTC Bit parameter info5/1(Flag)
  NTC Bit parameter info2/1(FltBit) -> Bitwise Operator/2
  NTC Bit parameter info3/1(FltBit) -> Bitwise Operator/3
  NTC Bit parameter info4/1(FltBit) -> Bitwise Operator/4
  NTC Bit parameter info5/1(FltBit) -> Bitwise Operator/5

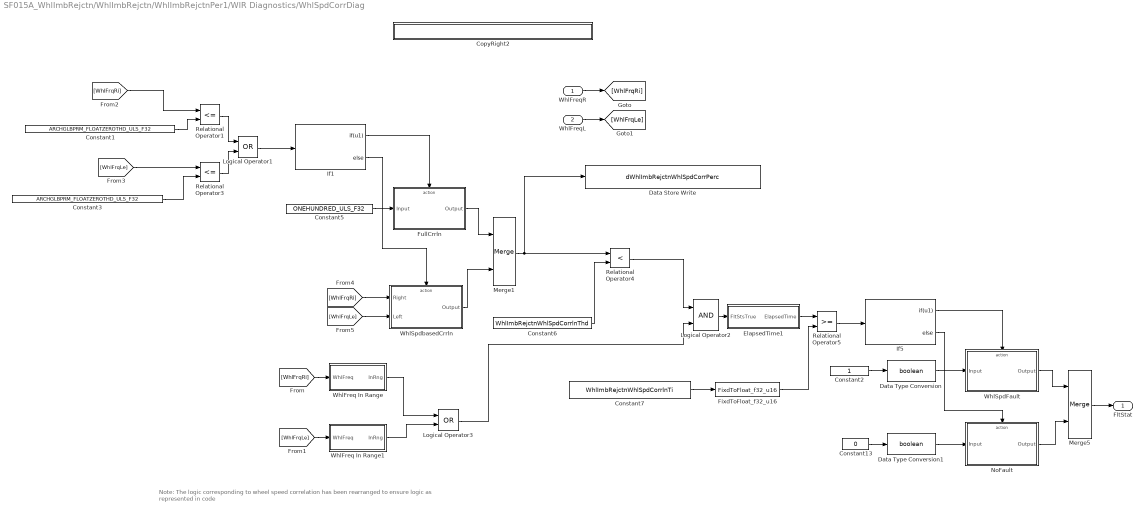
== system SF015A_WhlImbRejctn/WhlImbRejctn/WhlImbRejctnPer1/WIR Diagnostics/WhlSpdCorrDiag ==
  note: Note: The logic corresponding to wheel speed correlation has been rearranged to ensure logic as represented in code
  WhlFreqR : Inport
  WhlFreqL : Inport  Port=2
  Constant1 : Constant  Value=ARCHGLBPRM_FLOATZEROTHD_ULS_F32
  Constant13 : Constant  Value=0  OutDataTypeStr=boolean
  Constant2 : Constant  OutDataTypeStr=boolean
  Constant3 : Constant  Value=ARCHGLBPRM_FLOATZEROTHD_ULS_F32
  Constant5 : Constant  Value=ONEHUNDRED_ULS_F32
  Constant6 : Constant  Value=WhlImbRejctnWhlSpdCorrlnThd
  Constant7 : Constant  Value=WhlImbRejctnWhlSpdCorrlnTi
  CopyRight2 : Subsystem  Description=|  mask(Copyright Information){none=on}
      | Copyright info block.                                               
      |                                                                     
      | Place copyright information at the top of every subsystem in design.
      mask prompts: none "No parameters"
      mask help: Place copyright information at the top of every subsystem in design.
      mask Display:
      | NxtrConf = 'Nexteer Confidential';
      | 
      | sys = bdroot; %handle for the current model ("system")
      | first = get_param(sys,'Created');
      | first = first(end-3:end);  %year is last four digits
      | 
      | last = get_param(sys,'LastModifiedDate');
      | if isempty(last)
      |     last = datestr(now,'yyyy');
      | else
      |     last = last(end-3:end);
      | end
      | 
      | if strcmp(first,last)
      |     fprintf('%s -- Copyright %s Nexteer',NxtrConf,first)
      | else
      |     fprintf('%s -- %s%s- %s Nexteer',NxtrConf,char(169),first,last)
      | end
  Data Store Write : DataStoreWrite  DataStoreName=dWhlImbRejctnWhlSpdCorrPerc
  Data Type Conversion : DataTypeConversion  OutDataTypeStr=boolean
  Data Type Conversion1 : DataTypeConversion  OutDataTypeStr=boolean
  ElapsedTime1 : Subsystem  TreatAsAtomicUnit=on
  FixdToFloat_f32_u16 : FixdToFloat/FixdToFloat_f32_u16  Param1=0
  FullCrrln : Subsystem  RequirementInfo={} %GIDa_f316d04c_b5bf_4991_bd46_e1c3d0acec80  TreatAsAtomicUnit=on
  If1 : If  RequirementInfo={} %GIDa_4bc11ef0_d878_4cc4_82b4_0d0edb0129e4  IfExpression=u1
  If5 : If  RequirementInfo={} %GIDa_f8e2168d_295a_437f_93f0_d2de918d56ef  IfExpression=u1
  Logical Operator1 : Logic  Operator=OR  AllPortsSameDT=off  OutDataTypeStr=boolean
  Logical Operator2 : Logic  AllPortsSameDT=off  OutDataTypeStr=boolean
  Logical Operator3 : Logic  Operator=OR  AllPortsSameDT=off  OutDataTypeStr=boolean
  Merge1 : Merge
  Merge5 : Merge
  NoFault : Subsystem  RequirementInfo={} %GIDa_f7020847_ef3c_4257_9229_248ab4f76409  TreatAsAtomicUnit=on
  Relational Operator1 : RelationalOperator  Operator=<=  OutDataTypeStr=boolean
  Relational Operator3 : RelationalOperator  Operator=<=  OutDataTypeStr=boolean
  Relational Operator4 : RelationalOperator  Operator=<  OutDataTypeStr=boolean
  Relational Operator5 : RelationalOperator  OutDataTypeStr=boolean
  WhlFreq In Range : Subsystem
  WhlFreq In Range1 : Subsystem
  WhlSpdFault : Subsystem  RequirementInfo={} %GIDa_32897d14_0a36_471e_bba2_f76c6f004030  TreatAsAtomicUnit=on
  WhlSpdbasedCrrln : Subsystem  RequirementInfo={} %GIDa_bfd7bd1e_da2d_43b7_9815_cea994d6f624  TreatAsAtomicUnit=on
  FltStat : Outport
  wires:
  Merge5/1 -> FltStat/1
  Relational Operator1/1 -> Logical Operator1/1
  Relational Operator3/1 -> Logical Operator1/2
  Logical Operator1/1 -> If1/1
  Merge1/1 -> Data Store Write/1, Relational Operator4/1
  Constant6/1 -> Relational Operator4/2
  Constant7/1 -> FixdToFloat_f32_u16/1
  Relational Operator5/1 -> If5/1
  Relational Operator4/1 -> Logical Operator2/1
  WhlFreq In Range1/1(InRng) -> Logical Operator3/2
  WhlFreq In Range/1(InRng) -> Logical Operator3/1
  Logical Operator3/1 -> Logical Operator2/2
  If5/1 -> WhlSpdFault/Action
  If5/2 -> NoFault/Action
  WhlSpdFault/1(Output) -> Merge5/1
  NoFault/1(Output) -> Merge5/2
  Constant2/1 -> Data Type Conversion/1
  Constant13/1 -> Data Type Conversion1/1
  If1/1 -> FullCrrln/Action
  If1/2 -> WhlSpdbasedCrrln/Action
  FullCrrln/1(Output) -> Merge1/1
  WhlSpdbasedCrrln/1(Output) -> Merge1/2
  Constant5/1 -> FullCrrln/1(Input)
  ElapsedTime1/1(ElapsedTime) -> Relational Operator5/1
  Logical Operator2/1 -> ElapsedTime1/1(FltStsTrue)
  FixdToFloat_f32_u16/1 -> Relational Operator5/2
  Data Type Conversion/1 -> WhlSpdFault/1(Input)
  Data Type Conversion1/1 -> NoFault/1(Input)
  Constant3/1 -> Relational Operator3/2
  Constant1/1 -> Relational Operator1/2
  WhlFreqR/1 -> [WhlFrqRi]
  WhlFreqL/1 -> [WhlFrqLe]
  [WhlFrqRi] -> WhlFreq In Range/1(WhlFreq)
  [WhlFrqLe] -> WhlFreq In Range1/1(WhlFreq)
  [WhlFrqLe] -> Relational Operator3/1
  [WhlFrqRi] -> Relational Operator1/1
  [WhlFrqLe] -> WhlSpdbasedCrrln/2(Left)
  [WhlFrqRi] -> WhlSpdbasedCrrln/1(Right)

== system SF015A_WhlImbRejctn/WhlImbRejctn/WhlImbRejctnPer1/Whl Spd filter and Freq Estimation/CopyRight2 ==

== system SF015A_WhlImbRejctn/WhlImbRejctn/WhlImbRejctnPer1/Whl Spd filter and Freq Estimation/Tapped Delay Implementation ==
  Input : Inport
  Index : Inport  Port=2
  Tapped : Inport  Port=3
  Add1 : Sum
  Assignment : Assignment  IndexMode=Zero-based  IndexOptions=Index vector (port)  Indices=1  OutputSizes=128
  Constant : Constant  OutDataTypeStr=uint8
  Constant3 : Constant  Value=NROFDLY_CNT_U08
  CopyRight2 : Subsystem  Description=|  mask(Copyright Information){none=on}
      | Copyright info block.                                               
      |                                                                     
      | Place copyright information at the top of every subsystem in design.
      mask prompts: none "No parameters"
      mask help: Place copyright information at the top of every subsystem in design.
      mask Display:
      | NxtrConf = 'Nexteer Confidential';
      | 
      | sys = bdroot; %handle for the current model ("system")
      | first = get_param(sys,'Created');
      | first = first(end-3:end);  %year is last four digits
      | 
      | last = get_param(sys,'LastModifiedDate');
      | if isempty(last)
      |     last = datestr(now,'yyyy');
      | else
      |     last = last(end-3:end);
      | end
      | 
      | if strcmp(first,last)
      |     fprintf('%s -- Copyright %s Nexteer',NxtrConf,first)
      | else
      |     fprintf('%s -- %s%s- %s Nexteer',NxtrConf,char(169),first,last)
      | end
  If : If  IfExpression=u1
  If Action Subsystem : Subsystem  TreatAsAtomicUnit=on
  If Action Subsystem1 : Subsystem  TreatAsAtomicUnit=on
  Merge : Merge
  Relational Operator : RelationalOperator  OutDataTypeStr=boolean
  Tapped Signal : Outport
  Delay PIM : Outport  Port=2
  wires:
  Input/1 -> Assignment/2
  Index/1 -> Add1/1, Assignment/3
  Assignment/1 -> Tapped Signal/1
  Constant/1 -> Add1/2
  Add1/1 -> If Action Subsystem1/1(In1), Relational Operator/1
  Constant3/1 -> Relational Operator/2
  Relational Operator/1 -> If/1
  If/1 -> If Action Subsystem/Action
  If/2 -> If Action Subsystem1/Action
  Tapped/1 -> Assignment/1
  Merge/1 -> Delay PIM/1
  If Action Subsystem/1(Out1) -> Merge/1
  If Action Subsystem1/1(Out1) -> Merge/2

== system SF015A_WhlImbRejctn/WhlImbRejctn/WhlImbRejctnPer1/Whl Spd filter and Freq Estimation/Tapped Delay Implementation1 ==
  Input : Inport
  Index : Inport  Port=2
  Tapped : Inport  Port=3
  Add1 : Sum
  Assignment : Assignment  IndexMode=Zero-based  IndexOptions=Index vector (port)  Indices=1  OutputSizes=128
  Constant : Constant  OutDataTypeStr=uint8
  Constant3 : Constant  Value=NROFDLY_CNT_U08
  CopyRight2 : Subsystem  Description=|  mask(Copyright Information){none=on}
      | Copyright info block.                                               
      |                                                                     
      | Place copyright information at the top of every subsystem in design.
      mask prompts: none "No parameters"
      mask help: Place copyright information at the top of every subsystem in design.
      mask Display:
      | NxtrConf = 'Nexteer Confidential';
      | 
      | sys = bdroot; %handle for the current model ("system")
      | first = get_param(sys,'Created');
      | first = first(end-3:end);  %year is last four digits
      | 
      | last = get_param(sys,'LastModifiedDate');
      | if isempty(last)
      |     last = datestr(now,'yyyy');
      | else
      |     last = last(end-3:end);
      | end
      | 
      | if strcmp(first,last)
      |     fprintf('%s -- Copyright %s Nexteer',NxtrConf,first)
      | else
      |     fprintf('%s -- %s%s- %s Nexteer',NxtrConf,char(169),first,last)
      | end
  If : If  IfExpression=u1
  If Action Subsystem : Subsystem  TreatAsAtomicUnit=on
  If Action Subsystem1 : Subsystem  TreatAsAtomicUnit=on
  Merge : Merge
  Relational Operator : RelationalOperator  OutDataTypeStr=boolean
  Tapped Signal : Outport
  Delay PIM : Outport  Port=2
  wires:
  Input/1 -> Assignment/2
  Index/1 -> Add1/1, Assignment/3
  Assignment/1 -> Tapped Signal/1
  Constant/1 -> Add1/2
  Add1/1 -> If Action Subsystem1/1(In1), Relational Operator/1
  Constant3/1 -> Relational Operator/2
  Relational Operator/1 -> If/1
  If/1 -> If Action Subsystem/Action
  If/2 -> If Action Subsystem1/Action
  Tapped/1 -> Assignment/1
  Merge/1 -> Delay PIM/1
  If Action Subsystem/1(Out1) -> Merge/1
  If Action Subsystem1/1(Out1) -> Merge/2

== system SF015A_WhlImbRejctn/WhlImbRejctn/WhlImbRejctnPer1/Whl Spd filter and Freq Estimation/UGR L ==
  y : Inport
  FreqEst_Hz : Inport  Port=2
  PoleMag : Inport  Port=3
  Calc_ma1_a2 : Subsystem
  CopyRight2 : Subsystem  Description=|  mask(Copyright Information){none=on}
      | Copyright info block.                                               
      |                                                                     
      | Place copyright information at the top of every subsystem in design.
      mask prompts: none "No parameters"
      mask help: Place copyright information at the top of every subsystem in design.
      mask Display:
      | NxtrConf = 'Nexteer Confidential';
      | 
      | sys = bdroot; %handle for the current model ("system")
      | first = get_param(sys,'Created');
      | first = first(end-3:end);  %year is last four digits
      | 
      | last = get_param(sys,'LastModifiedDate');
      | if isempty(last)
      |     last = datestr(now,'yyyy');
      | else
      |     last = last(end-3:end);
      | end
      | 
      | if strcmp(first,last)
      |     fprintf('%s -- Copyright %s Nexteer',NxtrConf,first)
      | else
      |     fprintf('%s -- %s%s- %s Nexteer',NxtrConf,char(169),first,last)
      | end
  UnityGainResFilt : Subsystem
  y Filt : Outport
  wires:
  y/1 -> UnityGainResFilt/1(y)
  FreqEst_Hz/1 -> Calc_ma1_a2/1(f_est)
  UnityGainResFilt/1(Filt) -> y Filt/1
  Calc_ma1_a2/1(minus_a1) -> UnityGainResFilt/2(minus_a1)
  Calc_ma1_a2/2(a2) -> UnityGainResFilt/3(a2)
  PoleMag/1 -> Calc_ma1_a2/2(PoleMag)

== system SF015A_WhlImbRejctn/WhlImbRejctn/WhlImbRejctnPer1/Whl Spd filter and Freq Estimation/UGR R ==
  y : Inport
  FreqEst_Hz : Inport  Port=2
  PoleMag : Inport  Port=3
  Calc_ma1_a2 : Subsystem
  CopyRight2 : Subsystem  Description=|  mask(Copyright Information){none=on}
      | Copyright info block.                                               
      |                                                                     
      | Place copyright information at the top of every subsystem in design.
      mask prompts: none "No parameters"
      mask help: Place copyright information at the top of every subsystem in design.
      mask Display:
      | NxtrConf = 'Nexteer Confidential';
      | 
      | sys = bdroot; %handle for the current model ("system")
      | first = get_param(sys,'Created');
      | first = first(end-3:end);  %year is last four digits
      | 
      | last = get_param(sys,'LastModifiedDate');
      | if isempty(last)
      |     last = datestr(now,'yyyy');
      | else
      |     last = last(end-3:end);
      | end
      | 
      | if strcmp(first,last)
      |     fprintf('%s -- Copyright %s Nexteer',NxtrConf,first)
      | else
      |     fprintf('%s -- %s%s- %s Nexteer',NxtrConf,char(169),first,last)
      | end
  UnityGainResFilt : Subsystem
  y Filt : Outport
  wires:
  y/1 -> UnityGainResFilt/1(y)
  FreqEst_Hz/1 -> Calc_ma1_a2/1(f_est)
  UnityGainResFilt/1(Filt) -> y Filt/1
  Calc_ma1_a2/1(minus_a1) -> UnityGainResFilt/2(minus_a1)
  Calc_ma1_a2/2(a2) -> UnityGainResFilt/3(a2)
  PoleMag/1 -> Calc_ma1_a2/2(PoleMag)

== system SF015A_WhlImbRejctn/WhlImbRejctn/WhlImbRejctnPer2/Flt Recovery- DC Trend/CopyRight2 ==

== system SF015A_WhlImbRejctn/WhlImbRejctn/WhlImbRejctnPer2/Flt Recovery- DC Trend/ElapsedTime1 ==
  FltStsTrue : Inport
  CopyRight2 : Subsystem  Description=|  mask(Copyright Information){none=on}
      | Copyright info block.                                               
      |                                                                     
      | Place copyright information at the top of every subsystem in design.
      mask prompts: none "No parameters"
      mask help: Place copyright information at the top of every subsystem in design.
      mask Display:
      | NxtrConf = 'Nexteer Confidential';
      | 
      | sys = bdroot; %handle for the current model ("system")
      | first = get_param(sys,'Created');
      | first = first(end-3:end);  %year is last four digits
      | 
      | last = get_param(sys,'LastModifiedDate');
      | if isempty(last)
      |     last = datestr(now,'yyyy');
      | else
      |     last = last(end-3:end);
      | end
      | 
      | if strcmp(first,last)
      |     fprintf('%s -- Copyright %s Nexteer',NxtrConf,first)
      | else
      |     fprintf('%s -- %s%s- %s Nexteer',NxtrConf,char(169),first,last)
      | end
  Data Store Read : DataStoreRead  Priority=1  DataStoreName=DcTrendLrngEnaPrev
      settings: AttributesFormatString="priority:  %<Priority>"
  Data Store Write : DataStoreWrite  Priority=2  DataStoreName=DcTrendLrngEnaPrev
      settings: AttributesFormatString="priority:  %<Priority>"
  If : If  NumInputs=2  IfExpression=u1  ElseIfExpressions=u2
  If not true elapsed time = 0 : Subsystem  TreatAsAtomicUnit=on
  "If true and last step is true calculate elapsed time " : Subsystem  TreatAsAtomicUnit=on
  "If true and last step not true elapsed time = 0 get reference time " : Subsystem  TreatAsAtomicUnit=on
  Logical Operator1 : Logic  Operator=NOT  AllPortsSameDT=off  OutDataTypeStr=boolean
  Logical Operator2 : Logic  Operator=NOT  AllPortsSameDT=off  OutDataTypeStr=boolean
  Merge : Merge  Inputs=3
  ElapsedTime : Outport
  wires:
  If/1 -> If not true elapsed time = 0/Action
  If/2 -> "If true and last step not true elapsed time = 0 get reference time "/Action
  If/3 -> "If true and last step is true calculate elapsed time "/Action
  If not true elapsed time = 0/1(SpanTi) -> Merge/1
  "If true and last step not true elapsed time = 0 get reference time "/1("SpanTi ") -> Merge/2
  "If true and last step is true calculate elapsed time "/1(SpanTi) -> Merge/3
  Merge/1 -> ElapsedTime/1
  FltStsTrue/1 -> Logical Operator2/1, Data Store Write/1
  Data Store Read/1 -> Logical Operator1/1
  Logical Operator2/1 -> If/1
  Logical Operator1/1 -> If/2
